simulink model "AFCS_1(1)"  (R2016a)
settings: Solver=VariableStepAuto  StartTime=0.0  StopTime=200  RelTol=1e-3
values from neighbouring files (symbols this model uses):
  A = [ ... (first row only)    [AFCS.m]
  B = [ ... (first row only)    [AFCS.m]
  H1 = inv(B'*B)*B'*B1d    [AFCS.m]
  K1 = inv((B'*B))*B'*(A-A1d)    [AFCS.m]
settings Model: Creator=Administrator  LastModifiedBy=Administrator

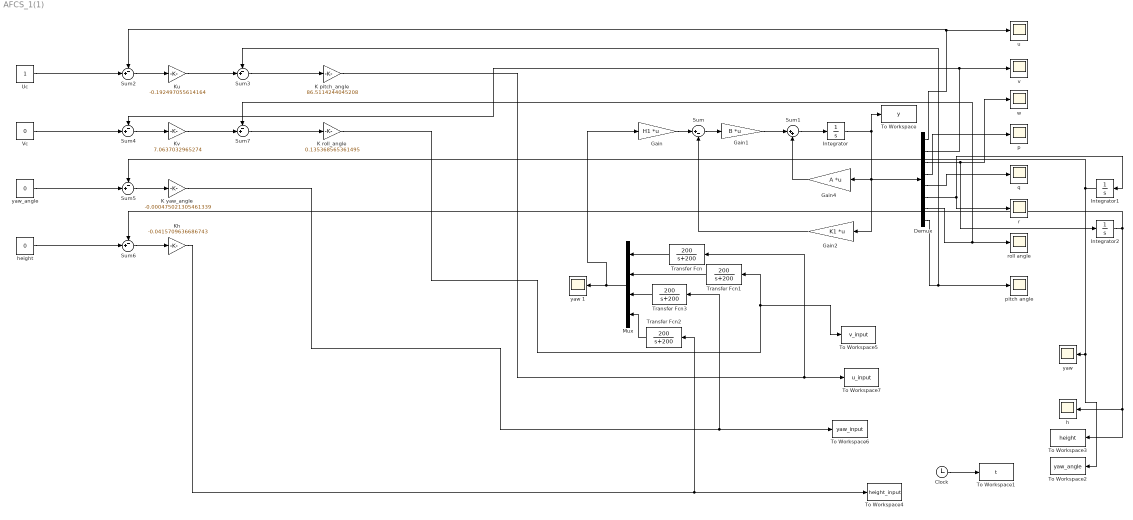
== system AFCS_1(1) ==
  Clock : Clock
  Demux : Demux  Outputs=8
  Gain : Gain  Gain=H1  Multiplication=Matrix(K*u)
  Gain1 : Gain  Gain=B  Multiplication=Matrix(K*u)
  Gain2 : Gain  Gain=K1  Multiplication=Matrix(K*u)
  Gain4 : Gain  Gain=A  Multiplication=Matrix(K*u)
  Integrator : Integrator
  Integrator1 : Integrator
  Integrator2 : Integrator
  "K pitch_angle " : Gain  Gain=86.5114244045208
  "K roll_angle " : Gain  Gain=0.135368565361495
  K yaw_angle : Gain  Gain=-0.000475021305461339
  Kh : Gain  Gain=-0.0415709636686743
  Ku : Gain  Gain=-0.192497055614164
  Kv : Gain  Gain=7.0637032965274
  Mux : Mux
  Sum : Sum  Inputs=|+-
  Sum1 : Sum  Inputs=|++
  Sum{2..7} (6 alike) : Sum  Inputs=-+|
  To Workspace : ToWorkspace  VariableName=y  SampleTime=-1
  To Workspace1 : ToWorkspace  VariableName=t  SampleTime=-1
  To Workspace2 : ToWorkspace  VariableName=yaw_angle  SampleTime=-1
  To Workspace3 : ToWorkspace  VariableName=height  SampleTime=-1
  To Workspace4 : ToWorkspace  VariableName=height_input  SampleTime=-1
  To Workspace5 : ToWorkspace  VariableName=v_input  SampleTime=-1
  To Workspace6 : ToWorkspace  VariableName=yaw_input  SampleTime=-1
  To Workspace7 : ToWorkspace  VariableName=u_input  SampleTime=-1
  Transfer Fcn{,1..3} (4 alike) : TransferFcn  Numerator=[200]  Denominator=[1 200]
  Uc : Constant
  Vc : Constant  Value=0
  h : Scope
  height : Constant  Value=0
  p : Scope
  pitch angle : Scope
  q : Scope
  r : Scope
  roll angle : Scope
  u : Scope
  v : Scope
  w : Scope
  "yaw " : Scope
  yaw 1 : Scope
  yaw_angle : Constant  Value=0
  wires:
  Mux/1 -> Gain/1, yaw 1/1
  Gain/1 -> Sum/1
  Sum/1 -> Gain1/1
  Sum1/1 -> Integrator/1
  Integrator/1 -> To Workspace/1, Gain2/1, Gain4/1, Demux/1
  Gain4/1 -> Sum1/2
  Gain2/1 -> Sum/2
  Gain1/1 -> Sum1/1
  Demux/2 -> v/1, Sum4/1
  Demux/3 -> Integrator2/1, w/1
  Demux/4 -> p/1
  Demux/5 -> q/1
  Demux/6 -> r/1, Integrator1/1
  Demux/7 -> Sum7/1, roll angle/1
  Sum2/1 -> Ku/1
  Sum3/1 -> "K pitch_angle "/1
  Demux/8 -> pitch angle/1, Sum3/1
  Demux/1 -> u/1, Sum2/1
  Clock/1 -> To Workspace1/1
  Ku/1 -> Sum3/2
  Integrator1/1 -> To Workspace2/1, "yaw "/1, Sum5/1
  Sum4/1 -> Kv/1
  Sum5/1 -> K yaw_angle/1
  Sum6/1 -> Kh/1
  Kv/1 -> Sum7/2
  Sum7/1 -> "K roll_angle "/1
  Integrator2/1 -> Sum6/1, To Workspace3/1, h/1
  height/1 -> Sum6/2
  Vc/1 -> Sum4/2
  Uc/1 -> Sum2/2
  yaw_angle/1 -> Sum5/2
  "K pitch_angle "/1 -> Transfer Fcn/1, To Workspace7/1
  "K roll_angle "/1 -> Transfer Fcn1/1, To Workspace5/1
  K yaw_angle/1 -> Transfer Fcn3/1, To Workspace6/1
  Kh/1 -> Transfer Fcn2/1, To Workspace4/1
  Transfer Fcn/1 -> Mux/1
  Transfer Fcn1/1 -> Mux/2
  Transfer Fcn3/1 -> Mux/3
  Transfer Fcn2/1 -> Mux/4
